simulink model "Xbox_controller"  (R2023a)
settings: Solver=VariableStepAuto  StartTime=0.0  StopTime=200  RelTol=1e-3
libraries: aerolibanimutils x2
settings Model: Creator=kaleb  LastModifiedBy=kaleb

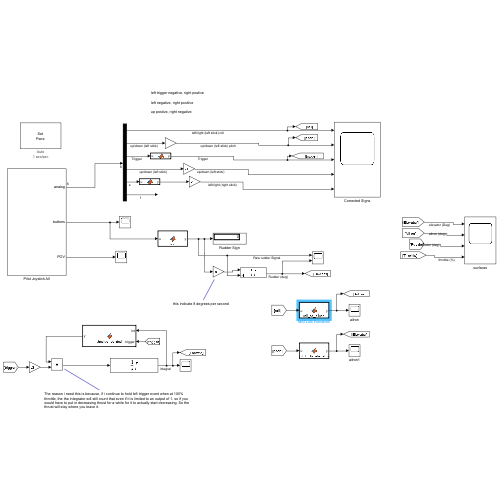
[thumbnail: Simulink's stored preview of the top-level diagram]
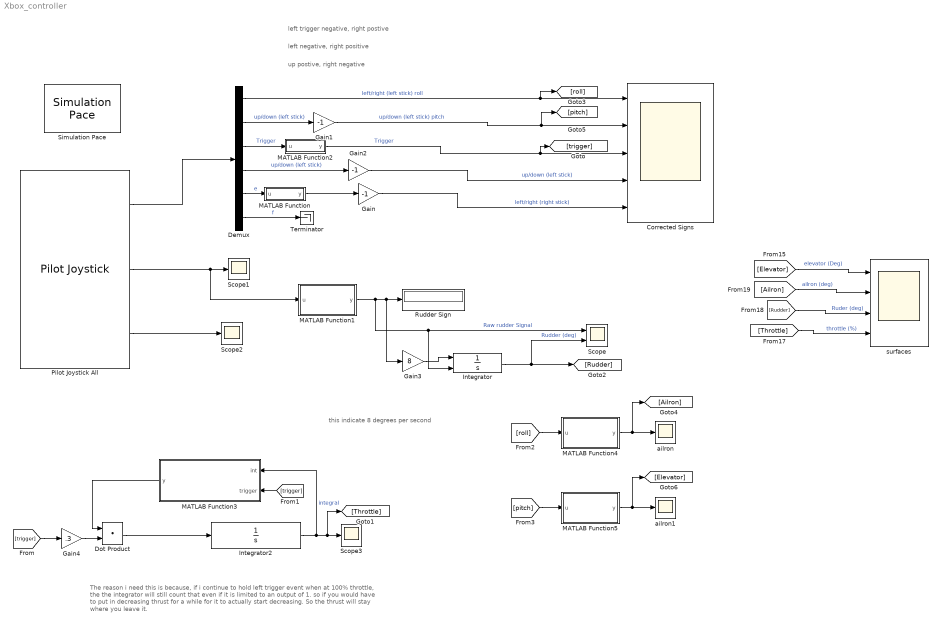
== system Xbox_controller ==
  note: The reason i need this is because, if i continue to hold left trigger event when at 100% throttle, the the integrator will still count that even if it is limited to an output of 1. so if you would have to put in decreasing thrust for a while for it to actually start decreasing. So the thrust will stay where you leave it.
  note: this indicate 8 degrees per second
  note: left trigger negative, right postive
  note: up postive, right negative
  note: left negative, right positive
  Corrected Signs : Scope  NumInputPorts=5
  Demux : Demux  Outputs=6
  Dot Product : DotProduct  OutDataTypeStr=Inherit: Inherit via internal rule
  Gain : Gain  Gain=-1
  Gain1 : Gain  Gain=-1
  Gain2 : Gain  Gain=-1
  Gain3 : Gain  Gain=8
  Gain4 : Gain  Gain=.3
  Integrator : Integrator  ExternalReset=either  LimitOutput=on  UpperSaturationLimit=30  LowerSaturationLimit=-30
  Integrator2 : Integrator  LimitOutput=on  UpperSaturationLimit=1  LowerSaturationLimit=0
  MATLAB Function : MATLAB Function  TreatAsAtomicUnit=on
  MATLAB Function1 : MATLAB Function  TreatAsAtomicUnit=on
  MATLAB Function2 : MATLAB Function  TreatAsAtomicUnit=on
  MATLAB Function3 : MATLAB Function  TreatAsAtomicUnit=on
  MATLAB Function4 : MATLAB Function  TreatAsAtomicUnit=on
  MATLAB Function5 : MATLAB Function  TreatAsAtomicUnit=on
  Pilot Joystick All : aerolibanimutils/Pilot Joystick  JoystickID=Joystick1  OutputConfiguration=AllOutputs  SampleTime=1/30
      settings: LibrarySourceBlock=aerolibanimutils/Pilot Joystick All
  Rudder Sign : Display
  Scope : Scope  NumInputPorts=2
  Scope1 : Scope
  Scope2 : Scope
  Scope3 : Scope
  Simulation Pace : aerolibanimutils/Simulation Pace  SimulationPace=1  SleepMode=Auto  OutputPaceError=off  SampleTime=1/30
  Terminator : Terminator
  ailron : Scope
  ailron1 : Scope
  surfaces : Scope  NumInputPorts=4
  wires:
  Pilot Joystick All/2 -> MATLAB Function1/1(u), Scope1/1
  Pilot Joystick All/3 -> Scope2/1
  Demux/1 -> [roll], Corrected Signs/1  "left/right (left stick) roll"
  Demux/2 -> Gain1/1  "up/down (left stick)"
  Demux/3 -> MATLAB Function2/1(u)  "Trigger"
  Demux/4 -> Gain2/1  "up/down (left stick)"
  Demux/6 -> Terminator/1  "f"
  Pilot Joystick All/1 -> Demux/1
  Gain/1 -> Corrected Signs/5  "left/right (right stick)"
  Demux/5 -> MATLAB Function/1(u)  "e"
  MATLAB Function/1(y) -> Gain/1
  Gain1/1 -> [pitch], Corrected Signs/2  "up/down (left stick) pitch"
  Gain2/1 -> Corrected Signs/4  "up/down (left stick)"
  MATLAB Function1/1(y) -> Integrator/2, Scope/1, Gain3/1, Rudder Sign/1  "Raw rudder Signal"
  Integrator/1 -> Scope/2, [Rudder]  "Rudder (deg)"
  Gain3/1 -> Integrator/1
  [trigger] -> Gain4/1
  Gain4/1 -> Dot Product/2
  Integrator2/1 -> MATLAB Function3/1(int), [Throttle], Scope3/1  "integral"
  MATLAB Function2/1(y) -> [trigger], Corrected Signs/3  "Trigger"
  Dot Product/1 -> Integrator2/1
  MATLAB Function3/1(y) -> Dot Product/1
  [trigger] -> MATLAB Function3/2(trigger)
  [roll] -> MATLAB Function4/1(u)
  MATLAB Function4/1(y) -> [Ailron], ailron/1
  MATLAB Function5/1(y) -> ailron1/1, [Elevator]
  [pitch] -> MATLAB Function5/1(u)
  [Ailron] -> surfaces/2  "ailron (deg)"
  [Elevator] -> surfaces/1  "elevator (Deg)"
  [Rudder] -> surfaces/3  "Ruder (deg)"
  [Throttle] -> surfaces/4  "throttle (%)"

== matlab function Xbox_controller/MATLAB Function ==
  data: u input; y output
function y = fcn(u)
%#codegen

y = u-.5;

== matlab function Xbox_controller/MATLAB Function2 ==
  data: u input; y output
function y = fcn(u)
%#codegen

y = u-.5;

== matlab function Xbox_controller/MATLAB Function3 ==
  data: int input; y output; trigger input
function y = throttle_control(int,trigger)
%#codegen

if int >= 1 && trigger >=0
y= 0;

elseif int <= 0 && trigger <=0
y= 0;

else
y=1;
end
end

== matlab function Xbox_controller/MATLAB Function4 ==
  data: u input; y output
function y = roll_to_ailron(u)
%this assumes that your max ailron is 25 deg
if sqrt(u^2) >= 0.08 %this is just the deadzone of my stick, and helps xbox stick drift

    y=-1*sign(u)*25*u^2;
else
    y=0;
end

end

== matlab function Xbox_controller/MATLAB Function5 ==
  data: u input; y output
function y = pitch_to_elevator(u)
%this assumes that your max ailron is 25 deg
if sqrt(u^2) >= 0.08 %this is just the deadzone of my stick, and helps xbox stick drift

    y=sign(u)*25*u^2;
else
    y=0;
end

end

== matlab function Xbox_controller/MATLAB Function1 ==
  data: u input; y output
function y = fcn(u)
%#codegen

if u == 16
y1;

elseif u == 32
y=-1;
elseif u == 48
y=0;
else
y=0;
end
end
